simulink model "Model2_Scenario1_Faulty_2020a"  (R2020b)
settings: Solver=FixedStepAuto  StartTime=0.0  StopTime=10.0  FixedStep=1e-3  RelTol=1e-3  EnableMultiTasking=on
undefined symbols (not defined in the file or in its folder): sigbuilder_block
settings Model: ExtModeTrigDuration=5  Creator=akshayjacob  LastModifiedBy=aarrieta
settings DataIOCC: SaveFormat=Array  SaveOutput=off  SaveTime=off  ReturnWorkspaceOutputs=off  SignalLoggingName=VRP_Test
settings OptimizationCC: DefaultParameterBehavior=Inlined  EnhancedBackFolding=on  PassReuseOutputArgsAs=Individual arguments  ZeroExternalMemoryAtStartup=off  ZeroInternalMemoryAtStartup=off  MaxStackSize=64  OptimizeBlockOrder=speed  DifferentSizesBufferReuse=on  OptimizationCustomize=off  EfficientTunableParamExpr=on
settings DebuggingCC: ParameterTunabilityLossMsg=error  SFMachineParentedDataDiag=error
settings HardwareCC: ProdBitPerPointer=32  ProdBitPerSizeT=32  ProdBitPerPtrDiffT=32  ProdLargestAtomicInteger=Long  ProdLargestAtomicFloat=Double  ProdWordSize=32  ProdHWDeviceType=ARM Compatible->ARM Cortex
settings SFSimCC: MATLABDynamicMemAlloc=off
settings RTWCC: Description=Embedded Coder  SystemTargetFile=ert.tlc  TemplateMakefile=ert_default_tmf  Toolchain=GNU Tools for ARM Embedded Processors
settings CodeAppCC: ForceParamTrailComments=on  IgnoreCustomStorageClasses=off  OperatorAnnotations=on  SimulinkDataObjDesc=on  SFDataObjDesc=on  InsertBlockDesc=on
settings ERTTargetCC: ERTCustomFileTemplate=example_file_process.tlc

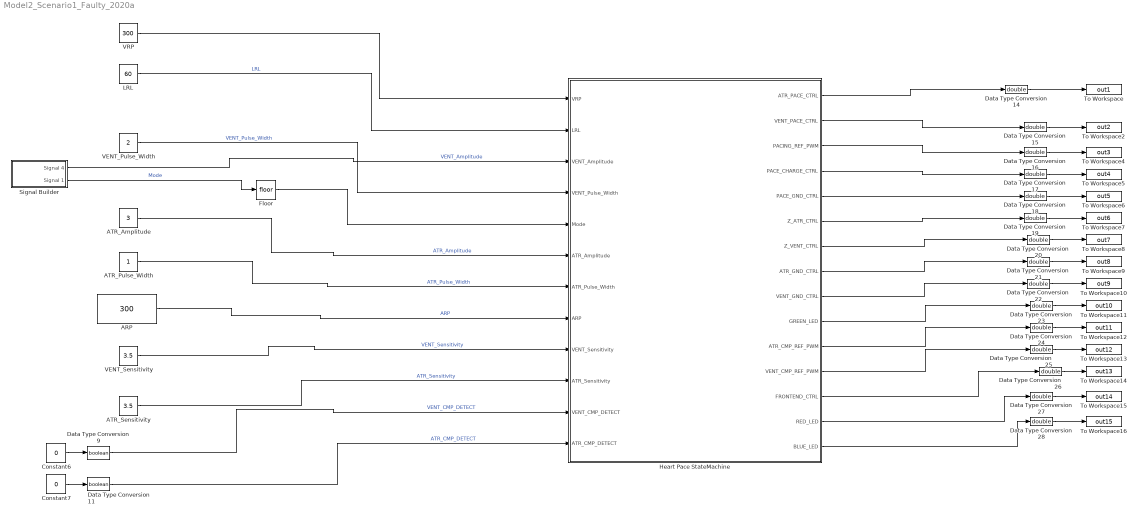
== system Model2_Scenario1_Faulty_2020a ==
  ARP : Constant  Value=300  OutDataTypeStr=uint16
  ATR_Amplitude : Constant  Value=3
  ATR_Pulse_Width : Constant
  ATR_Sensitivity : Constant  Value=3.5
  Constant6 : Constant  Value=0
  Constant7 : Constant  Value=0
  Data Type Conversion11 : DataTypeConversion  OutDataTypeStr=boolean
  Data Type Conversion{14..28} (15 alike) : DataTypeConversion  OutDataTypeStr=double
  Data Type Conversion9 : DataTypeConversion  OutDataTypeStr=boolean
  Floor : Rounding
  Heart Pace StateMachine : Stateflow chart  TreatAsAtomicUnit=on
      settings: PortSchema="{\"entries\":[{\"content\":{\"sides\":[{\"content\":{\"connectorIds\":[\"In1\",\"In2\",\"In3\",\"In4\",\"In5\",\"In6\",\"In7\",\"In8\",\"In9\",\"In10\",\"In11\",\"In12\"]},\"type\":\"ConnectorPlacement.EquallySpacedRectSide\",\"uuid\":\"078f44e2-9792-46c6-9fab-c05fe0916fc5\"},{\"content\":{\"connectorIds\":[\"Out1\",\"Out2\",\"Out3\",\"Out4\",\"Out5\",\"Out6\",\"Out7\",\"Out8\",\"Out9\",\"Out13\",\"Out14\",\"Out15\",\"Out10\",\"Out11\",\"Out12\"],\"side\":\"RIGHT\"},\"type\":\"ConnectorPlacement.EquallySpacedRectSide\",\"uuid\":\"2df68980-2ea6-42d1-b726-b24978220bfa\"},{\"content\":{\"connectorIds\":[],\"side\":\"TOP\"},\"type\":\"ConnectorPlacement.EquallySpacedRectSide\",\"uuid\":\"4f99418a-e276-4e4c-8fb0-96ffb017fecf\"}]},\"type\":\"ConnectorPlacement.EquallySpacedConnector\",\"uuid\":\"ac4267e7-732c-486f-b9a5-28cca0f40ec4\"}],\"packageUris\":[\"http://schema.mathworks.com/mf0/Connector/R2020b\"],\"version\":\"1.0\"}"
  LRL : Constant  Value=60
  Signal Builder : Subsystem  Tag=STV Subsys  LoadFcn=sigbuilder_block('load');  StartFcn=sigbuilder_block('start');  StopFcn=sigbuilder_block('stop');  ClipboardFcn=sigbuilder_block('clipboard');  mask(Sigbuilder block){tuvar=[0:10]}
      mask help: Simulink:masks:SigbuilderBlock_MD
      mask init:
      | if ~strcmp(get_param(bdroot(gcbh),'SimulationStatus'),'stopped') tuvar = sigbuilder_block('maskInit'); end
      settings: CopyFcn=sigbuilder_block('copy');  DeleteFcn=sigbuilder_block('delete');  ModelCloseFcn=sigbuilder_block('modelClose');  PreSaveFcn=sigbuilder_block('preSave');  PauseFcn=sigbuilder_block('pause');  ContinueFcn=sigbuilder_block('continue');  NameChangeFcn=sigbuilder_block('namechange');  OpenFcn=sigbuilder_block('open',[6 26.4 948 559.8 ]);  CloseFcn=sigbuilder_block('close');
      mask Display: plot(0, 0, 100, 100,[2, 2, 32, 32, 2], [68, 8, 8, 68, 68],[32, 2], [38, 38], [32, 19, 2],[53, 60, 44], [32, 17, 17, 2],[16, 16, 31, 31]);txt = getActiveGroup(gcbh);text(2, 100, txt,'verticalAlignment', 'top');
  To Workspace : ToWorkspace  VariableName=out1  SaveFormat=Timeseries  SampleTime=-1
  To Workspace10 : ToWorkspace  VariableName=out9  SaveFormat=Timeseries  SampleTime=-1
  To Workspace11 : ToWorkspace  VariableName=out10  SaveFormat=Timeseries  SampleTime=-1
  To Workspace12 : ToWorkspace  VariableName=out11  SaveFormat=Timeseries  SampleTime=-1
  To Workspace13 : ToWorkspace  VariableName=out12  SaveFormat=Timeseries  SampleTime=-1
  To Workspace14 : ToWorkspace  VariableName=out13  SaveFormat=Timeseries  SampleTime=-1
  To Workspace15 : ToWorkspace  VariableName=out14  SaveFormat=Timeseries  SampleTime=-1
  To Workspace16 : ToWorkspace  VariableName=out15  SaveFormat=Timeseries  SampleTime=-1
  To Workspace2 : ToWorkspace  VariableName=out2  SaveFormat=Timeseries  SampleTime=-1
  To Workspace4 : ToWorkspace  VariableName=out3  SaveFormat=Timeseries  SampleTime=-1
  To Workspace5 : ToWorkspace  VariableName=out4  SaveFormat=Timeseries  SampleTime=-1
  To Workspace6 : ToWorkspace  VariableName=out5  SaveFormat=Timeseries  SampleTime=-1
  To Workspace7 : ToWorkspace  VariableName=out6  SaveFormat=Timeseries  SampleTime=-1
  To Workspace8 : ToWorkspace  VariableName=out7  SaveFormat=Timeseries  SampleTime=-1
  To Workspace9 : ToWorkspace  VariableName=out8  SaveFormat=Timeseries  SampleTime=-1
  VENT_Pulse_Width : Constant  Value=2
  VENT_Sensitivity : Constant  Value=3.5
  VRP : Constant  Value=300
  wires:
  ARP/1 -> Heart Pace StateMachine/8(ARP)  "ARP"
  VENT_Sensitivity/1 -> Heart Pace StateMachine/9(VENT_Sensitivity)  "VENT_Sensitivity"
  Data Type Conversion11/1 -> Heart Pace StateMachine/12(ATR_CMP_DETECT)  "ATR_CMP_DETECT"
  VENT_Pulse_Width/1 -> Heart Pace StateMachine/4(VENT_Pulse_Width)  "VENT_Pulse_Width"
  Signal Builder/2(Signal 1) -> Floor/1  "Mode"
  ATR_Pulse_Width/1 -> Heart Pace StateMachine/7(ATR_Pulse_Width)  "ATR_Pulse_Width"
  LRL/1 -> Heart Pace StateMachine/2(LRL)  "LRL"
  ATR_Sensitivity/1 -> Heart Pace StateMachine/10(ATR_Sensitivity)  "ATR_Sensitivity"
  Signal Builder/1(Signal 4) -> Heart Pace StateMachine/3(VENT_Amplitude)  "VENT_Amplitude"
  Data Type Conversion9/1 -> Heart Pace StateMachine/11(VENT_CMP_DETECT)  "VENT_CMP_DETECT"
  ATR_Amplitude/1 -> Heart Pace StateMachine/6(ATR_Amplitude)  "ATR_Amplitude"
  VRP/1 -> Heart Pace StateMachine/1(VRP)
  Constant7/1 -> Data Type Conversion11/1
  Constant6/1 -> Data Type Conversion9/1
  Floor/1 -> Heart Pace StateMachine/5(Mode)
  Data Type Conversion23/1 -> To Workspace11/1
  Data Type Conversion26/1 -> To Workspace14/1
  Data Type Conversion25/1 -> To Workspace13/1
  Data Type Conversion27/1 -> To Workspace15/1
  Data Type Conversion22/1 -> To Workspace10/1
  Data Type Conversion28/1 -> To Workspace16/1
  Data Type Conversion14/1 -> To Workspace/1
  Data Type Conversion21/1 -> To Workspace9/1
  Data Type Conversion16/1 -> To Workspace4/1
  Data Type Conversion17/1 -> To Workspace5/1
  Data Type Conversion15/1 -> To Workspace2/1
  Data Type Conversion24/1 -> To Workspace12/1
  Data Type Conversion18/1 -> To Workspace6/1
  Data Type Conversion20/1 -> To Workspace8/1
  Data Type Conversion19/1 -> To Workspace7/1
  Heart Pace StateMachine/1(ATR_PACE_CTRL) -> Data Type Conversion14/1
  Heart Pace StateMachine/2(VENT_PACE_CTRL) -> Data Type Conversion15/1
  Heart Pace StateMachine/3(PACING_REF_PWM) -> Data Type Conversion16/1
  Heart Pace StateMachine/4(PACE_CHARGE_CTRL) -> Data Type Conversion17/1
  Heart Pace StateMachine/5(PACE_GND_CTRL) -> Data Type Conversion18/1
  Heart Pace StateMachine/6(Z_ATR_CTRL) -> Data Type Conversion19/1
  Heart Pace StateMachine/7(Z_VENT_CTRL) -> Data Type Conversion20/1
  Heart Pace StateMachine/8(ATR_GND_CTRL) -> Data Type Conversion21/1
  Heart Pace StateMachine/9(VENT_GND_CTRL) -> Data Type Conversion22/1
  Heart Pace StateMachine/13(GREEN_LED) -> Data Type Conversion23/1
  Heart Pace StateMachine/14(ATR_CMP_REF_PWM) -> Data Type Conversion24/1
  Heart Pace StateMachine/15(VENT_CMP_REF_PWM) -> Data Type Conversion25/1
  Heart Pace StateMachine/10(FRONTEND_CTRL) -> Data Type Conversion26/1
  Heart Pace StateMachine/11(RED_LED) -> Data Type Conversion27/1
  Heart Pace StateMachine/12(BLUE_LED) -> Data Type Conversion28/1

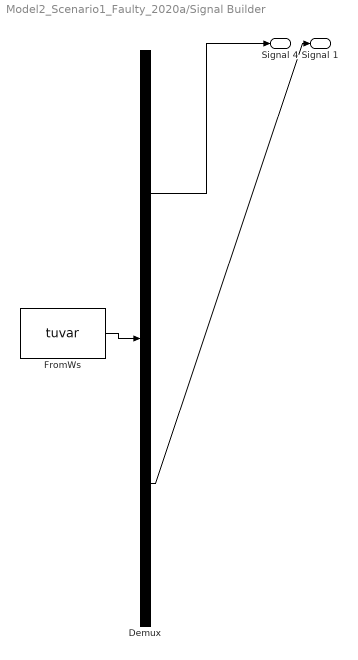
== system Model2_Scenario1_Faulty_2020a/Signal Builder ==
  Demux : Demux  Tag=STV Demux  Outputs=2
      settings: DisplayOption=none
  FromWs : FromWorkspace  Tag=STV FromWs  VariableName=tuvar
      SigBuilderData=|
      | common.afterFinalStr = 'Extrapolate'
      | common.sampleTime = 0
      | dataSet(1).timeRange = [0 300]
      | dataSet(1).name = 'Group 1'
      | dataSet(2).timeRange = [0 300]
      | dataSet(2).name = 'Group 2'
      | sbobj.Groups(1).Name = 'Group 1'
      | sbobj.Groups(1).Signals(1).Name = 'Signal 4'
      | sbobj.Groups(1).Signals(1).XData = [0 16.5 16.5 39.5 39.5 102 102 207 207 254.5 254.5 300]
      | sbobj.Groups(1).Signals(1).YData = [0 0 15 15 20 20 10 10 30 30 0 0]
      | sbobj.Groups(1).Signals(2).Name = 'Signal 1'
      | sbobj.Groups(1).Signals(2).XData = [0 10.5 50.5 50.5 81.5 81.5 140.5 140.5 182.5 182.5 244.5 244.5 300]
      | sbobj.Groups(1).Signals(2).YData = [2 2 2 3 3 4 4 2 2 1 1 0 0]
      | sbobj.Groups(1).TimeRange = [0 300]
      | sbobj.Groups(2).Name = 'Group 2'
      | sbobj.Groups(2).Signals(1).Name = 'Signal 4'
      | sbobj.Groups(2).Signals(1).XData = [0 16.5 16.5 39.5 39.5 102 102 207 254.5 300]
      | sbobj.Groups(2).Signals(1).YData = [0 0 15 15 20 20 0 0 0 0]
      | sbobj.Groups(2).Signals(2).Name = 'Signal 1'
      | sbobj.Groups(2).Signals(2).XData = [0 10.5 10.5 50.5 50.5 81.5 81.5 140.5 140.5 182.5 182.5 244.5 244.5 300]
      | sbobj.Groups(2).Signals(2).YData = [0 0 0 0 3 3 0 0 2 2 1 1 2 2]
      | sbobj.Groups(2).TimeRange = [0 300]
  Signal 4 : Outport  Tag=STV Outport
  Signal 1 : Outport  Tag=STV Outport  Port=2
  wires:
  FromWs/1 -> Demux/1
  Demux/1 -> Signal 4/1
  Demux/2 -> Signal 1/1

== stateflow chart Model2_Scenario1_Faulty_2020a/Heart Pace StateMachine ==
  state VOO_ChargingState
    entry:
    ATR_PACE_CTRL = 0;
    VENT_PACE_CTRL = 0;
    PACING_REF_PWM = VENT_Amplitude/5*100
    PACE_CHARGE_CTRL = 1;
    PACE_GND_CTRL = 1;
    Z_ATR_CTRL = 0;
    Z_VENT_CTRL = 0;
    ATR_GND_CTRL = 0;
    VENT_GND_CTRL = 1;
    BLUE_LED = 0;
    RED_LED = 1;
  state VOO_Pacing
    entry:
    PACE_CHARGE_CTRL = 0;
    PACE_GND_CTRL = 1;
    ATR_GND_CTRL = 0;
    ATR_PACE_CTRL = 0;
    Z_ATR_CTRL = 0;
    Z_VENT_CTRL =0;
    VENT_PACE_CTRL = 1;
    VENT_GND_CTRL = 0;
    PACING_REF_PWM = VENT_Amplitude/5*100;
    BLUE_LED=1;
    RED_LED=0;
  state AOO_ChargingState
    entry:
    ATR_PACE_CTRL = 0;
    VENT_PACE_CTRL = 0;
    PACING_REF_PWM = ATR_Amplitude/5*100
    PACE_CHARGE_CTRL = 1;
    PACE_GND_CTRL = 1;
    Z_ATR_CTRL = 0;
    Z_VENT_CTRL = 0;
    ATR_GND_CTRL = 1;
    VENT_GND_CTRL = 0;
    BLUE_LED = 0;
    RED_LED = 1;
  state AOO_Pacing
    entry:
    PACE_CHARGE_CTRL = 0;
    PACE_GND_CTRL = 1;
    ATR_GND_CTRL = 0;
    ATR_PACE_CTRL = 1;
    Z_ATR_CTRL = 0;
    Z_VENT_CTRL =0;
    VENT_PACE_CTRL = 0;
    VENT_GND_CTRL = 0;
    PACING_REF_PWM = ATR_Amplitude/5*100;
    BLUE_LED=1;
    RED_LED=0;
  state MAIN
    entry:
    PACE_CHARGE_CTRL = 0;
    VENT_PACE_CTRL = 0;
    ATR_PACE_CTRL = 0;
    PACE_GND_CTRL = 0;
    ATR_GND_CTRL = 0;
    VENT_GND_CTRL = 0;
    Z_ATR_CTRL = 0;
    Z_VENT_CTRL = 0;
    FRONTEND_CTRL = 0;
    RED_LED = 0;
    BLUE_LED=0;
    Flag = 0;
  state VVI_Sensing
    entry:
    BLUE_LED = 0;
    RED_LED = 0;
    GREEN_LED = 1;
    Flag = 0;
  state VVI_Refactory
    entry:
    ATR_PACE_CTRL = 0;
    VENT_PACE_CTRL = 0;
    PACING_REF_PWM = VENT_Amplitude/5*100;
    PACE_CHARGE_CTRL = 1;
    PACE_GND_CTRL = 1;
    Z_ATR_CTRL = 0;
    Z_VENT_CTRL = 0;
    ATR_GND_CTRL = 0;
    VENT_GND_CTRL = 1;
    FRONTEND_CTRL = 1;
    VENT_CMP_REF_PWM = 125;
    BLUE_LED = 0;
    RED_LED = 1;
    GREEN_LED = 0;
  state VVI_Pacing
    entry:
    FRONTEND_CTRL = 0;
    PACE_CHARGE_CTRL = 0;
    PACE_GND_CTRL = 1;
    ATR_GND_CTRL = 0;
    ATR_PACE_CTRL = 0;
    Z_ATR_CTRL = 0;
    Z_VENT_CTRL =0;
    VENT_PACE_CTRL = 1;
    VENT_GND_CTRL = 0;
    PACING_REF_PWM = VENT_Amplitude/5*100;
    BLUE_LED = 1;
    RED_LED = 0;
    GREEN_LED = 0;
    Flag = 1;
  state AAI_Sensing
    entry:
    BLUE_LED = 0;
    RED_LED = 0;
    GREEN_LED = 1;
    Flag = 0;
  note: Subtract PW from this based on previous event
      | -sense heart rate: dont (no pulsewith done by pacemaker)
      | -pulsed rate: subtract PW
      |  vrp-(pulsewith*flag)
  state AAI_Refactory
    entry:
    ATR_PACE_CTRL = 0;
    VENT_PACE_CTRL = 0;
    PACING_REF_PWM = ATR_Amplitude/5*100;
    PACE_CHARGE_CTRL = 1;
    PACE_GND_CTRL = 1;
    Z_ATR_CTRL = 0;
    Z_VENT_CTRL = 0;
    ATR_GND_CTRL = 1;
    VENT_GND_CTRL = 0;
    FRONTEND_CTRL = 1;
    ATR_CMP_REF_PWM= ATR_Sensitivity/5*100;
    BLUE_LED = 0;
    RED_LED = 1;
    GREEN_LED = 1;
  state AAI_Pacing
    entry:
    FRONTEND_CTRL = 0;
    PACE_CHARGE_CTRL = 0;
    PACE_GND_CTRL = 1;
    ATR_GND_CTRL = 0;
    ATR_PACE_CTRL = 1;
    Z_ATR_CTRL = 0;
    Z_VENT_CTRL =0;
    VENT_PACE_CTRL = 0;
    VENT_GND_CTRL = 0;
    PACING_REF_PWM = ATR_Amplitude/5*100;
    BLUE_LED = 1;
    RED_LED = 0;
    GREEN_LED = 0;
    Flag = 1;
  VOO_ChargingState -> VOO_Pacing : after((60000/LRL) - VENT_Pulse_Width,msec)
  MAIN -> VOO_ChargingState [order 1] : [Mode == 0]
  VOO_Pacing -> VOO_ChargingState : after(VENT_Pulse_Width, msec)
  (default) -> MAIN
  AOO_ChargingState -> AOO_Pacing : after((60000/LRL) - ATR_Pulse_Width,msec)
  MAIN -> AOO_ChargingState [order 4] : [Mode == 1]
  AOO_Pacing -> AOO_ChargingState : after(ATR_Pulse_Width, msec)
  MAIN -> VVI_Refactory [order 2] : [Mode == 2]
  MAIN -> AAI_Refactory [order 3] : [Mode==3]
  VVI_Refactory -> VVI_Sensing : after(VRP - (VENT_Pulse_Width * Flag),msec)
  VVI_Sensing -> VVI_Pacing [order 2] : after(60000/LRL - VRP, msec)
  VVI_Sensing -> VVI_Refactory [order 1] : [(VENT_CMP_DETECT == 1)]
  VVI_Pacing -> VVI_Refactory : after(VENT_Pulse_Width,msec)
  AAI_Refactory -> AAI_Sensing : after(ARP  - (ATR_Pulse_Width * Flag),msec)
  AAI_Sensing -> AAI_Pacing [order 2] : after(60000/LRL - ARP, msec)
  AAI_Sensing -> AAI_Refactory [order 1] : [ATR_CMP_DETECT == 1]
  AAI_Pacing -> AAI_Refactory : after(ATR_Pulse_Width,msec)
  data: VRP input; LRL input; VENT_Amplitude input; VENT_Pulse_Width input; Mode input; ATR_PACE_CTRL output; VENT_PACE_CTRL output; PACING_REF_PWM output; PACE_CHARGE_CTRL output; PACE_GND_CTRL output; Z_ATR_CTRL output; Z_VENT_CTRL output; ATR_GND_CTRL output; VENT_GND_CTRL output; FRONTEND_CTRL output; RED_LED output =0; BLUE_LED output; ATR_Amplitude input; ATR_Pulse_Width input; ARP input; VENT_Sensitivity input; ATR_Sensitivity input; GREEN_LED output; VENT_CMP_DETECT input; ATR_CMP_DETECT input; Flag local; ATR_CMP_REF_PWM output; VENT_CMP_REF_PWM output
